simulink library "shared_library"  (R2022a)
settings: Solver=VariableStepAuto  StartTime=0.0  StopTime=10.0  RelTol=1e-3
settings Model: Creator=KenYoshioka  LastModifiedBy=KenYoshioka

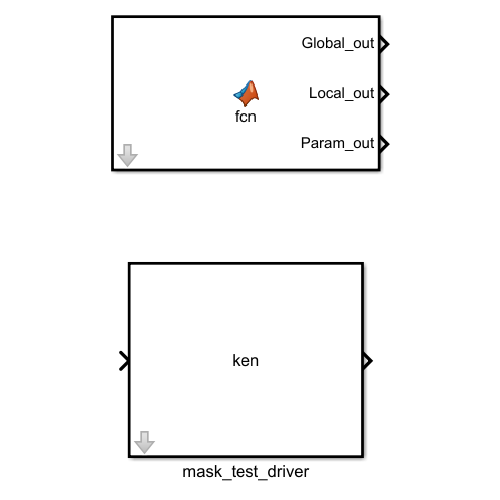
[thumbnail: Simulink's stored preview of the top-level diagram]
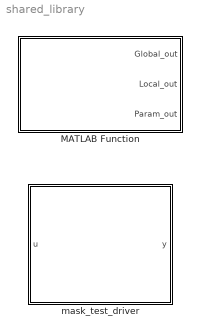
== system shared_library ==
  MATLAB Function : MATLAB Function  TreatAsAtomicUnit=on  mask{Param_test=0}
      mask init:
      | global Global_test;
      | 
      | if (~evalin('base','mask_initialized'))
      |     evalin('base','mask_initialized=1;');
      |     Global_test = 1;
      |     Param_test = 2;
      | end
      | 
      | Local_test = evalin('base','Local_test');
      | 
      | Global_test = Global_test + 10;
      | Local_test = Local_test + 10;
      | Param_test = Global_test;
      | 
      | assignin('base','Local_test',Local_test);
  mask_test_driver : MATLAB Function  TreatAsAtomicUnit=on  mask{Param_init=0}
      mask init:
      | maskObj = MaskTest(gcb);

== matlab function shared_library/mask_test_driver ==
  data: u input; y output
function y = fcn(u)

y = u;

== matlab function shared_library/MATLAB Function ==
  data: Global_out output; Global_test parameter; Local_test parameter; Param_test parameter; Local_out output; Param_out output
function [Global_out,Local_out,Param_out] = fcn(Global_test, Local_test, Param_test)
Global_out = Global_test;
Local_out = Local_test;
Param_out = Param_test;
